simulink model "lagrange"  (R2018b)
settings: Solver=VariableStepAuto  StartTime=0.0  StopTime=3  RelTol=1e-3
settings Model: Creator=dongdaming  LastModifiedBy=dongdaming

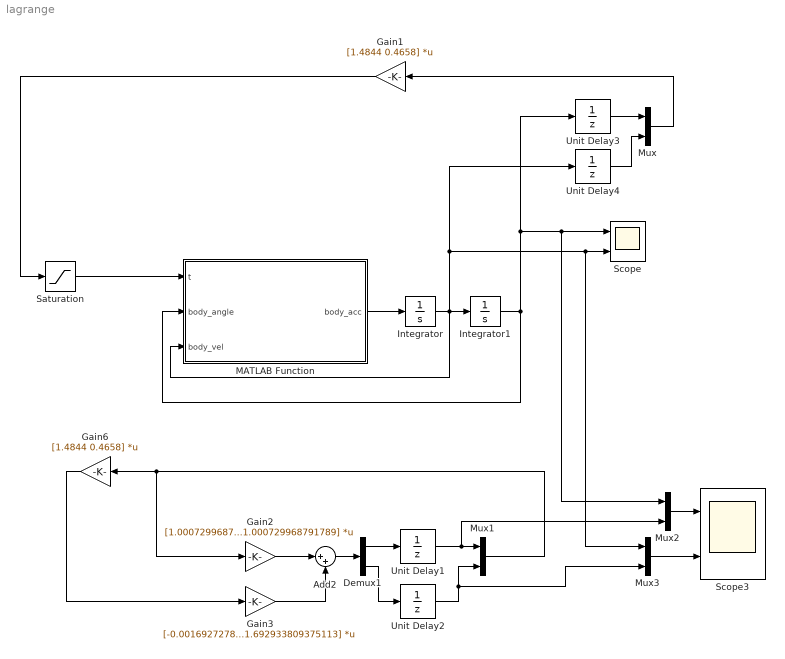
== system lagrange ==
  Add2 : Sum  Inputs=|++
  Demux1 : Demux  Outputs=2
  Gain1 : Gain  Gain=[1.4844 0.4658]  Multiplication=Matrix(K*u)
  Gain2 : Gain  Gain=[1.000729968791789,0.002000486622183;0.730057587899423,1.000729968791789]  Multiplication=Matrix(K*u)
  Gain3 : Gain  Gain=[-0.001692727899678;-1.692933809375113]  Multiplication=Matrix(K*u)
  Gain6 : Gain  Gain=[1.4844 0.4658]  Multiplication=Matrix(K*u)
  Integrator : Integrator
  Integrator1 : Integrator  InitialCondition=pi/3  LimitOutput=on  UpperSaturationLimit=pi  LowerSaturationLimit=-pi
  MATLAB Function : MATLAB Function  TreatAsAtomicUnit=on
  Mux{,1..3} (4 alike) : Mux  Inputs=2
  Saturation : Saturate  UpperLimit=1.4  LowerLimit=-1.4
  Scope : Scope  NumInputPorts=2
  Scope3 : Scope  NumInputPorts=2
  Unit Delay1 : UnitDelay  InitialCondition=pi/3  SampleTime=-1
  Unit Delay2 : UnitDelay  SampleTime=-1
  Unit Delay3 : UnitDelay  InitialCondition=pi/3  SampleTime=0.002
  Unit Delay4 : UnitDelay  InitialCondition=pi/3  SampleTime=0.002
  wires:
  MATLAB Function/1(body_acc) -> Integrator/1
  Integrator/1 -> Mux3/1, Scope/2, Unit Delay4/1, MATLAB Function/3(body_vel), Integrator1/1
  Integrator1/1 -> Unit Delay3/1, Mux2/1, Scope/1, MATLAB Function/2(body_angle)
  Saturation/1 -> MATLAB Function/1(t)
  Gain1/1 -> Saturation/1
  Gain3/1 -> Add2/2
  Gain2/1 -> Add2/1
  Add2/1 -> Demux1/1
  Demux1/1 -> Unit Delay1/1
  Mux1/1 -> Gain2/1, Gain6/1
  Unit Delay1/1 -> Mux2/2, Mux1/1
  Demux1/2 -> Unit Delay2/1
  Unit Delay2/1 -> Mux1/2, Mux3/2
  Gain6/1 -> Gain3/1
  Unit Delay3/1 -> Mux/1
  Unit Delay4/1 -> Mux/2
  Mux/1 -> Gain1/1
  Mux2/1 -> Scope3/1
  Mux3/1 -> Scope3/2

== matlab function lagrange/MATLAB Function ==
  data: t input; body_acc output; body_angle input; body_vel input
function body_acc = fcn(t,body_angle,body_vel)
body_acc=(+1429.48*sin(body_angle)-1215.55*t-2083.85*t*cos(body_angle)-3.87597*sin(2*body_angle)*body_vel^2)/(2.91931+cos(body_angle)^2+8.75194*sin(body_angle)^2);
